simulink model "F16_dynamic_model_2019a"  (R2024b)
settings: Solver=ode3  StartTime=0.0  StopTime=1  FixedStep=1/1000  RelTol=1e-3
values from neighbouring files (symbols this model uses):
  f16data =     [f16aerodata.mat]
  f16engine =     [f16engine.mat]
undefined symbols (not defined in the file or in its folder): e0_0, e1_0, e2_0, e3_0, Earth, ft, m, s, WGS84
libraries: simulink_extras x11, simulink x7, aerosimlib x5, vrlib x3, sharedtransform x3, aerolibfltsims x3, slpidlib x3, aerolibconvert2 x2, aerolibutil x1, sharedutil x1, shared6dof x1, aerolibtransform2 x1
(part 3 of 3)

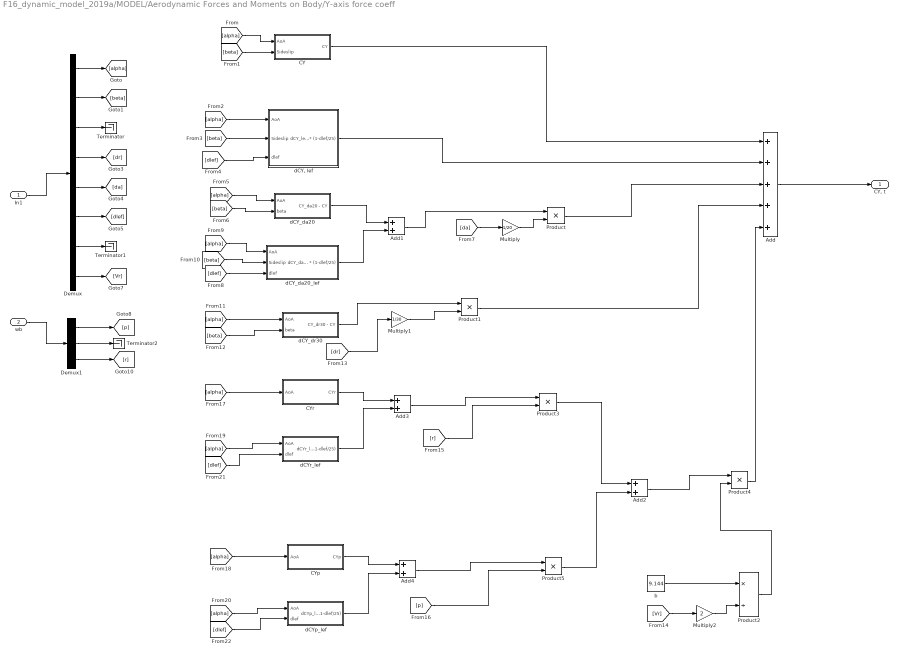
== system F16_dynamic_model_2019a/MODEL/Aerodynamic Forces and Moments on Body/Y-axis force coeff ==
  In1 : Inport
  "wb " : Inport  Port=2
  Add : Sum  Inputs=+++++
  Add{1..4} (4 alike) : Sum
  CY : Subsystem
  CYp : Subsystem
  CYr : Subsystem
  Demux : Demux  Outputs=8
  Demux1 : Demux  Outputs=3
  Multiply : Gain  Gain=1/20
  Multiply1 : Gain  Gain=1/30
  Multiply2 : Gain  Gain=2
  Product{,1,3..5} (5 alike) : Product
  Product2 : Product  Inputs=*/
  Terminator : Terminator
  Terminator1 : Terminator
  Terminator2 : Terminator
  b : Constant  Value=9.144
  "dCY, lef " : Subsystem
  dCY_da20 : Subsystem
  dCY_da20_lef : Subsystem
  dCY_dr30 : Subsystem
  dCYp_lef : Subsystem
  dCYr_lef : Subsystem
  "CY, t" : Outport
  wires:
  Demux/3 -> Terminator/1
  Demux/1 -> [alpha]
  Demux/7 -> Terminator1/1
  Demux/8 -> [Vr]
  Demux/6 -> [dlef]
  Demux/4 -> [dr]
  Demux/2 -> [beta]
  Demux/5 -> [da]
  In1/1 -> Demux/1
  "wb "/1 -> Demux1/1
  Demux1/1 -> [p]
  Demux1/2 -> Terminator2/1
  Demux1/3 -> [r]
  [alpha] -> CY/1(AoA)
  [beta] -> CY/2("Sideslip ")
  Add/1 -> "CY, t"/1
  CY/1(CY) -> Add/1
  [dlef] -> "dCY, lef "/3(dlef)
  [beta] -> "dCY, lef "/2("Sideslip ")
  [alpha] -> "dCY, lef "/1(AoA)
  "dCY, lef "/1(dCY_lef * (1-dlef/25)) -> Add/2
  [alpha] -> dCY_da20/1(AoA)
  [beta] -> dCY_da20/2(beta)
  dCY_da20/1(CY_da20 - CY) -> Add1/1
  Add1/1 -> Product/1
  Product/1 -> Add/3
  [da] -> Multiply/1
  Multiply/1 -> Product/2
  [dlef] -> dCY_da20_lef/3(dlef)
  [beta] -> dCY_da20_lef/2("Sideslip ")
  [alpha] -> dCY_da20_lef/1(AoA)
  dCY_da20_lef/1(dCY_da20lef * (1-dlef/25)) -> Add1/2
  [alpha] -> dCY_dr30/1(AoA)
  [beta] -> dCY_dr30/2(beta)
  dCY_dr30/1(CY_dr30 - CY) -> Product1/1
  [dr] -> Multiply1/1
  Multiply1/1 -> Product1/2
  Product1/1 -> Add/4
  [Vr] -> Multiply2/1
  b/1 -> Product2/1
  Multiply2/1 -> Product2/2
  [r] -> Product3/2
  Product3/1 -> Add2/1
  Add2/1 -> Product4/1
  Product2/1 -> Product4/2
  Product4/1 -> Add/5
  [p] -> Product5/2
  Product5/1 -> Add2/2
  [alpha] -> CYr/1(AoA)
  [alpha] -> dCYr_lef/1(AoA)
  CYr/1(CYr) -> Add3/1
  dCYr_lef/1(dCYr_lef * (1-dlef/25)) -> Add3/2
  Add3/1 -> Product3/1
  CYp/1("CYp ") -> Add4/1
  dCYp_lef/1(dCYp_lef * (1-dlef/25)) -> Add4/2
  Add4/1 -> Product5/1
  [alpha] -> CYp/1(AoA)
  [alpha] -> dCYp_lef/1(AoA)
  [dlef] -> dCYr_lef/2(dlef)
  [dlef] -> dCYp_lef/2(dlef)

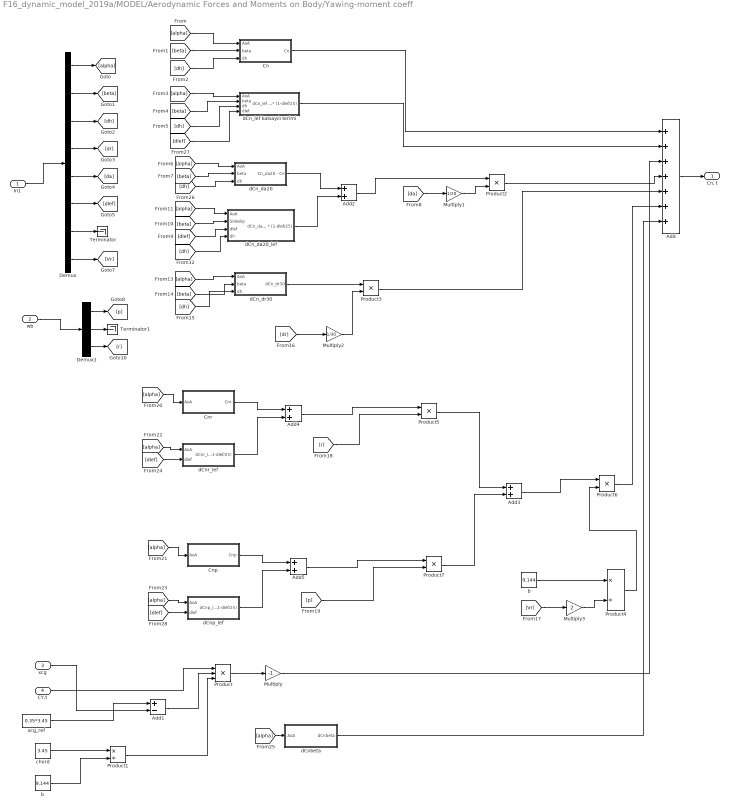
== system F16_dynamic_model_2019a/MODEL/Aerodynamic Forces and Moments on Body/Yawing-moment coeff ==
  In1 : Inport
  wb : Inport  Port=2
  xcg : Inport  Port=3
  CY,t : Inport  Port=4
  Add : Sum  Inputs=+++++++
  Add1 : Sum  Inputs=+-
  Add{2..5} (4 alike) : Sum
  Cn : Subsystem
  Cnp : Subsystem
  Cnr : Subsystem
  Demux : Demux  Outputs=8
  Demux1 : Demux  Outputs=3
  Multiply : Gain  Gain=-1
  Multiply1 : Gain  Gain=1/20
  Multiply2 : Gain  Gain=1/30
  Multiply3 : Gain  Gain=2
  Product : Product  Inputs=3
  Product1 : Product  Inputs=*/
  Product{2..3,5..7} (5 alike) : Product
  Product4 : Product  Inputs=*/
  Terminator : Terminator
  Terminator1 : Terminator
  b : Constant  Value=9.144
  "b " : Constant  Value=9.144
  chord : Constant  Value=3.45
  dCn_da20 : Subsystem
  dCn_da20_lef : Subsystem
  dCn_dr30 : Subsystem
  dCn_lef katsayılı terimi : Subsystem
  dCnbeta : Subsystem
  dCnp_lef : Subsystem
  dCnr_lef : Subsystem
  xcg_ref : Constant  Value=0.35*3.45
  "Cn, t" : Outport
  wires:
  Demux/3 -> [dh]
  Demux/1 -> [alpha]
  Demux/7 -> Terminator/1
  Demux/8 -> [Vr]
  Demux/6 -> [dlef]
  Demux/4 -> [dr]
  Demux/2 -> [beta]
  Demux/5 -> [da]
  In1/1 -> Demux/1
  wb/1 -> Demux1/1
  Demux1/1 -> [p]
  Demux1/2 -> Terminator1/1
  Demux1/3 -> [r]
  [alpha] -> Cn/1(AoA)
  [beta] -> Cn/2("beta ")
  [dh] -> Cn/3(dh)
  [alpha] -> dCn_lef katsayılı terimi/1(AoA)
  [beta] -> dCn_lef katsayılı terimi/2(beta)
  [dh] -> dCn_lef katsayılı terimi/3(dh)
  Cn/1(Cn) -> Add/1
  dCn_lef katsayılı terimi/1(dCn_lef * (1-dlef/25)) -> Add/2
  CY,t/1 -> Product/1
  xcg_ref/1 -> Add1/1
  xcg/1 -> Add1/2
  Add1/1 -> Product/2
  chord/1 -> Product1/1
  "b "/1 -> Product1/2
  Product1/1 -> Product/3
  Product/1 -> Multiply/1
  Multiply/1 -> Add/3
  Add/1 -> "Cn, t"/1
  Add2/1 -> Product2/1
  [beta] -> dCn_da20_lef/2("Sideslip ")
  dCn_da20_lef/1(dCn_da20lef * (1-dlef/25)) -> Add2/2
  dCn_da20/1(Cn_da20 - Cn) -> Add2/1
  [alpha] -> dCn_da20_lef/1(AoA)
  Product2/1 -> Add/4
  Multiply1/1 -> Product2/2
  [da] -> Multiply1/1
  [alpha] -> dCn_da20/1(AoA)
  [dlef] -> dCn_da20_lef/3(dlef)
  [beta] -> dCn_da20/2(beta)
  [dh] -> dCn_da20_lef/4(dh)
  [alpha] -> dCn_dr30/1(AoA)
  [beta] -> dCn_dr30/2(beta)
  [dh] -> dCn_dr30/3(dh)
  [dr] -> Multiply2/1
  Multiply2/1 -> Product3/2
  dCn_dr30/1(dCn_dr30) -> Product3/1
  Product3/1 -> Add/5
  b/1 -> Product4/1
  Product7/1 -> Add3/2
  Add3/1 -> Product6/1
  [alpha] -> dCnp_lef/1(AoA)
  [alpha] -> Cnp/1(AoA)
  Add5/1 -> Product7/1
  Cnp/1("Cnp ") -> Add5/1
  dCnp_lef/1(dCnp_lef * (1-dlef/25)) -> Add5/2
  dCnr_lef/1(dCnr_lef * (1-dlef/25)) -> Add4/2
  [Vr] -> Multiply3/1
  Multiply3/1 -> Product4/2
  Cnr/1(Cnr) -> Add4/1
  Add4/1 -> Product5/1
  [alpha] -> Cnr/1(AoA)
  [alpha] -> dCnr_lef/1(AoA)
  Product6/1 -> Add/6
  [r] -> Product5/2
  [p] -> Product7/2
  Product5/1 -> Add3/1
  Product4/1 -> Product6/2
  [dlef] -> dCnr_lef/2(dlef)
  [alpha] -> dCnbeta/1(AoA)
  dCnbeta/1("dCnbeta ") -> Add/7
  [dh] -> dCn_da20/3(dh)
  [dlef] -> dCn_lef katsayılı terimi/4(dlef)
  [dlef] -> dCnp_lef/2(dlef)

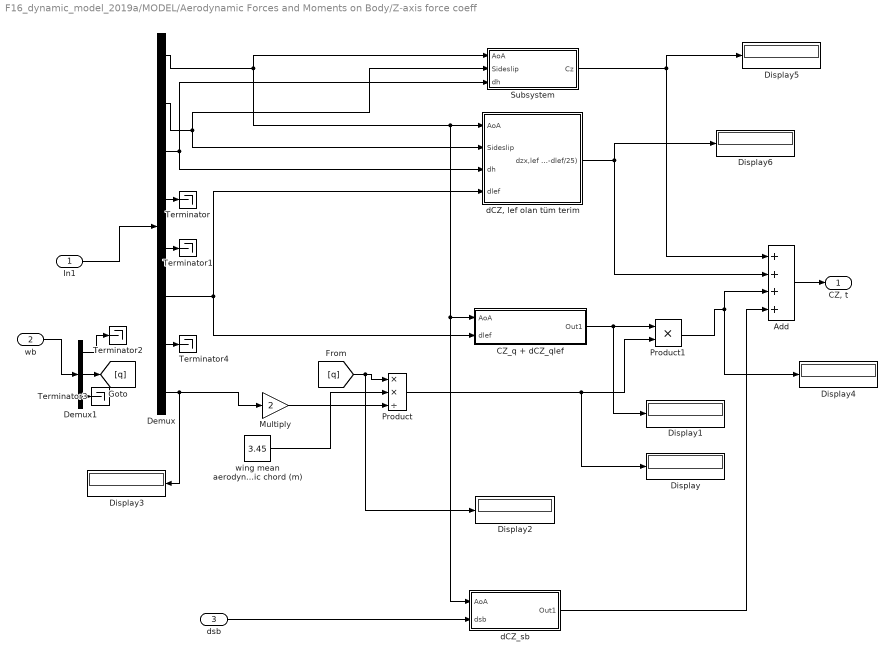
== system F16_dynamic_model_2019a/MODEL/Aerodynamic Forces and Moments on Body/Z-axis force coeff ==
  In1 : Inport
  wb : Inport  Port=2
  dsb : Inport  Port=3
  Add : Sum  Inputs=++++
  CZ_q + dCZ_qlef : Subsystem
  Demux : Demux  Outputs=8
  Demux1 : Demux  Outputs=3
  Display{,1..6} (7 alike) : Display
  Multiply : Gain  Gain=2
  Product : Product  Inputs=**/
  Product1 : Product
  Subsystem : Subsystem
  Terminator{,1..4} (5 alike) : Terminator
  "dCZ, lef olan tüm terim" : Subsystem
  dCZ_sb : Subsystem
  wing mean aerodynamic chord (m) : Constant  Value=3.45
  "CZ, t" : Outport
  wires:
  Product1/1 -> Display4/1, Add/3
  Product/1 -> Display/1, Product1/2
  Multiply/1 -> Product/3
  wing mean aerodynamic chord (m)/1 -> Product/2
  Demux/8 -> Multiply/1, Display3/1
  Demux/5 -> Terminator1/1
  Demux/4 -> Terminator/1
  CZ_q + dCZ_qlef/1(Out1) -> Display1/1, Product1/1
  Demux/6 -> "dCZ, lef olan tüm terim"/4(dlef), CZ_q + dCZ_qlef/2(dlef)
  Demux/3 -> Subsystem/3(dh), "dCZ, lef olan tüm terim"/3(dh)
  Demux/2 -> "dCZ, lef olan tüm terim"/2("Sideslip "), Subsystem/2(Sideslip)
  Demux/1 -> Subsystem/1(AoA), "dCZ, lef olan tüm terim"/1(AoA), dCZ_sb/1(AoA), CZ_q + dCZ_qlef/1(AoA)
  "dCZ, lef olan tüm terim"/1(dzx,lef * (1-dlef/25)) -> Add/2, Display6/1
  Subsystem/1(Cz) -> Add/1, Display5/1
  Add/1 -> "CZ, t"/1
  In1/1 -> Demux/1
  Demux1/2 -> [q]
  Demux1/1 -> Terminator2/1
  wb/1 -> Demux1/1
  Demux1/3 -> Terminator3/1
  [q] -> Display2/1, Product/1
  Demux/7 -> Terminator4/1
  dsb/1 -> dCZ_sb/2(dsb)
  dCZ_sb/1(Out1) -> Add/4

== system F16_dynamic_model_2019a/MODEL/Thrust on Body /Subsystem ==
  Mil : Inport
  Idle : Inport  Port=2
  power : Inport  Port=3
  Max : Inport  Port=4
  Display : Display
  Display1 : Display
  Display2 : Display
  Multiply : Gain  Gain=4.448
  Subsystem : Subsystem
  Subsystem1 : Subsystem
  Switch : Switch  Criteria=u2 > Threshold  Threshold=50  SaturateOnIntegerOverflow=off  InputSameDT=off
  Thrust : Outport
  wires:
  Mil/1 -> [T_Mil]
  Idle/1 -> [T_Idle]
  [T_Mil] -> Subsystem/1(mil)
  [T_Max] -> Subsystem/2("max ")
  Max/1 -> [T_Max]
  power/1 -> Display2/1, [Power]
  [Power] -> Subsystem/3(power)
  Subsystem/1(T) -> Display/1, Switch/1
  [Power] -> Switch/2
  [T_Mil] -> Subsystem1/1("Mil ")
  Subsystem1/1(T) -> Switch/3, Display1/1
  Switch/1 -> Multiply/1
  [T_Idle] -> Subsystem1/2(Idle)
  [Power] -> Subsystem1/3(Power)
  Multiply/1 -> Thrust/1

== system F16_dynamic_model_2019a/MODEL/gravity/gravity_body_axis ==
  gravity : Inport
  "phi theta psi " : Inport  Port=2
  Demux : Demux  Outputs=3
  Gain : Gain  Gain=-1
  Mux : Mux  Inputs=3
  Product : Product
  Product1 : Product
  Product2 : Product
  SinCos : Trigonometry  Operator=sincos
  SinCos1 : Trigonometry  Operator=sincos
  Terminator : Terminator
  gravity_body : Outport
  wires:
  Demux/1 -> SinCos/1
  Demux/2 -> SinCos1/1
  SinCos/1 -> Product/1
  SinCos1/2 -> Product/2, Product1/2
  Product/1 -> Mux/2
  SinCos/2 -> Product1/1
  Product1/1 -> Mux/3
  SinCos1/1 -> Gain/1
  Gain/1 -> Mux/1
  gravity/1 -> Product2/1
  Mux/1 -> Product2/2
  Product2/1 -> gravity_body/1
  "phi theta psi "/1 -> Demux/1
  Demux/3 -> Terminator/1

== system F16_dynamic_model_2019a/MODEL/6-DOF Model Body Euler/Subsystem/Subsystem ==
  p q r : Inport
  q0 q1 q2 q3 : Inport  Port=2
  Constant : Constant
  Dot Product : DotProduct  InputSameDT=off  OutDataTypeStr=Inherit: Inherit via internal rule
  High Gain Quaternion Normalization : Gain  SaturateOnIntegerOverflow=on  OutDataTypeStr=Inherit: Same as input  ParamDataTypeStr=Inherit: Same as input
  Mux1 : Mux  Inputs=[3 4 1]
  Mux2 : Mux
  Sum : Sum  Inputs=|+-  InputSameDT=on  SaturateOnIntegerOverflow=on  OutDataTypeStr=Inherit: Same as first input
  q0dot : Fcn  Expr=-0.5 * ( u[5]*u[1]+u[6]*u[2]+u[7]*u[3] ) + u[8]*u[4]
  q1dot : Fcn  Expr=0.5 * ( u[4]*u[1]+u[6]*u[3]-u[7]*u[2] ) + u[8]*u[5]
  q2dot : Fcn  Expr=0.5 * ( u[4]*u[2]+u[7]*u[1]-u[5]*u[3] ) + u[8]*u[6]
  q3dot : Fcn  Expr=0.5 * ( u[4]*u[3]+u[5]*u[2]-u[6]*u[1] ) + u[8]*u[7]
  qdot : Outport  InitialOutput=0  VectorParamsAs1DForOutWhenUnconnected=off
  wires:
  q0 q1 q2 q3/1 -> Dot Product/1, Dot Product/2, Mux1/2
  q3dot/1 -> Mux2/4
  Mux2/1 -> qdot/1
  Mux1/1 -> q2dot/1, q3dot/1, q0dot/1, q1dot/1
  Sum/1 -> High Gain Quaternion Normalization/1
  q1dot/1 -> Mux2/2
  Dot Product/1 -> Sum/2
  High Gain Quaternion Normalization/1 -> Mux1/3
  q0dot/1 -> Mux2/1
  Constant/1 -> Sum/1
  p q r/1 -> Mux1/1
  q2dot/1 -> Mux2/3

== system F16_dynamic_model_2019a/MODEL/Aerodynamic Forces and Moments on Body/Pitching-moment coeff/Cm ==
  AoA : Inport
  beta : Inport  Port=2
  dh : Inport  Port=3
  n-D Lookup Table : Lookup_n-D  NumberOfTableDimensions=3  BreakpointsForDimension1=f16data.alpha1  BreakpointsForDimension2=f16data.beta  BreakpointsForDimension3=f16data.de1  Table=f16data.Cm  InterpMethod=Cubic spline  ExtrapMethod=Clip  InternalRulePriority=Speed  RndMeth=Simplest
      settings: InputPortMap=u0,u1,u2
  Cm : Outport
  wires:
  n-D Lookup Table/1 -> Cm/1
  beta/1 -> n-D Lookup Table/2
  AoA/1 -> n-D Lookup Table/1
  dh/1 -> n-D Lookup Table/3

== system F16_dynamic_model_2019a/MODEL/Aerodynamic Forces and Moments on Body/Pitching-moment coeff/Cm_q - dCm_qlef ==
  AoA : Inport
  dlef : Inport  Port=2
  Add : Sum
  Cmq : Lookup_n-D  NumberOfTableDimensions=1  BreakpointsForDimension1=f16data.alpha1  BreakpointsForDimension3=[5, 7]  Table=f16data.Cmq  ExtrapMethod=Clip  InternalRulePriority=Speed  RndMeth=Simplest
  Constant : Constant
  Display : Display
  Multiply : Gain  Gain=1/(25)
  Product : Product
  Sum : Sum  Inputs=+-
  dCmq_lef : Lookup_n-D  NumberOfTableDimensions=1  BreakpointsForDimension1=f16data.alpha2  BreakpointsForDimension3=[5, 7]  Table=f16data.dCmq_lef  ExtrapMethod=Clip  InternalRulePriority=Speed  RndMeth=Simplest
  Out1 : Outport
  wires:
  Multiply/1 -> Sum/2
  Constant/1 -> Sum/1
  Sum/1 -> Product/2
  dlef/1 -> Multiply/1
  Product/1 -> Add/2
  AoA/1 -> Cmq/1, dCmq_lef/1
  Cmq/1 -> Display/1, Add/1
  dCmq_lef/1 -> Product/1
  Add/1 -> Out1/1

== system F16_dynamic_model_2019a/MODEL/Aerodynamic Forces and Moments on Body/Pitching-moment coeff/dCm ==
  AoA : Inport
  n-D Lookup Table : Lookup_n-D  NumberOfTableDimensions=1  BreakpointsForDimension1=f16data.alpha1  BreakpointsForDimension3=[5, 7]  Table=f16data.dCm  ExtrapMethod=Clip  InternalRulePriority=Speed  RndMeth=Simplest
  dCm : Outport
  wires:
  n-D Lookup Table/1 -> dCm/1
  AoA/1 -> n-D Lookup Table/1

== system F16_dynamic_model_2019a/MODEL/Aerodynamic Forces and Moments on Body/Pitching-moment coeff/dCm, lef olan tüm terim ==
  AoA : Inport
  "Sideslip " : Inport  Port=2
  dh : Inport  Port=3
  dlef : Inport  Port=4
  Cm : Lookup_n-D  NumberOfTableDimensions=3  BreakpointsForDimension1=f16data.alpha1  BreakpointsForDimension2=f16data.beta  BreakpointsForDimension3=f16data.de1  Table=f16data.Cm  ExtrapMethod=Clip  InternalRulePriority=Speed  RndMeth=Simplest
      settings: InputPortMap=u0,u1,u2
  Cm_lef : Lookup_n-D  BreakpointsForDimension1=f16data.alpha2  BreakpointsForDimension2=f16data.beta  BreakpointsForDimension3=[5, 7]  Table=f16data.Cm_lef  ExtrapMethod=Clip  InternalRulePriority=Speed  RndMeth=Simplest
      settings: InputPortMap=u0,u1
  Constant : Constant
  Multiply : Gain  Gain=1/(25)
  Multiply1 : Gain  Gain=0
  Product : Product
  Sum : Sum  Inputs=+-
  dcm,lef : Sum  Inputs=+-
  dcm,lef * (1-dlef/25) : Outport
  wires:
  dlef/1 -> Multiply/1
  Multiply/1 -> Sum/2
  Constant/1 -> Sum/1
  Sum/1 -> Product/2
  dh/1 -> Multiply1/1
  dcm,lef/1 -> Product/1
  Product/1 -> dcm,lef * (1-dlef/25)/1
  Cm/1 -> dcm,lef/2
  Cm_lef/1 -> dcm,lef/1
  AoA/1 -> Cm/1, Cm_lef/1
  "Sideslip "/1 -> Cm/2, Cm_lef/2
  Multiply1/1 -> Cm/3

== system F16_dynamic_model_2019a/MODEL/Aerodynamic Forces and Moments on Body/Pitching-moment coeff/dCm_ds ==
  AoA : Inport
  dh : Inport  Port=2
  n-D Lookup Table : Lookup_n-D  BreakpointsForDimension1=f16data.alpha1  BreakpointsForDimension2=f16data.de3  BreakpointsForDimension3=[5, 7]  Table=f16data.dCm_ds  ExtrapMethod=Clip  InternalRulePriority=Speed  RndMeth=Simplest
      settings: InputPortMap=u0,u1
  dCm_ds : Outport
  wires:
  n-D Lookup Table/1 -> dCm_ds/1
  dh/1 -> n-D Lookup Table/2
  AoA/1 -> n-D Lookup Table/1

== system F16_dynamic_model_2019a/MODEL/Aerodynamic Forces and Moments on Body/Pitching-moment coeff/dCm_sb ==
  AoA : Inport
  dsb : Inport  Port=2
  Multiply : Gain  Gain=1/60
  Product : Product
  n-D Lookup Table : Lookup_n-D  NumberOfTableDimensions=1  BreakpointsForDimension1=f16data.alpha1  BreakpointsForDimension3=[5, 7]  Table=f16data.dCm_sb  ExtrapMethod=Clip  InternalRulePriority=Speed  RndMeth=Simplest
  Out1 : Outport
  wires:
  dsb/1 -> Multiply/1
  AoA/1 -> n-D Lookup Table/1
  n-D Lookup Table/1 -> Product/1
  Multiply/1 -> Product/2
  Product/1 -> Out1/1

== system F16_dynamic_model_2019a/MODEL/Aerodynamic Forces and Moments on Body/Rolling-moment coeff/Cl ==
  AoA : Inport
  "beta " : Inport  Port=2
  dh : Inport  Port=3
  Cl table : Lookup_n-D  NumberOfTableDimensions=3  BreakpointsForDimension1=f16data.alpha1  BreakpointsForDimension2=f16data.beta  BreakpointsForDimension3=f16data.de2  Table=f16data.Cl  ExtrapMethod=Clip  InternalRulePriority=Speed  RndMeth=Simplest
      settings: InputPortMap=u0,u1,u2
  Cl : Outport
  wires:
  AoA/1 -> Cl table/1
  "beta "/1 -> Cl table/2
  dh/1 -> Cl table/3
  Cl table/1 -> Cl/1

== system F16_dynamic_model_2019a/MODEL/Aerodynamic Forces and Moments on Body/Rolling-moment coeff/Clp ==
  AoA : Inport
  Clp : Lookup_n-D  NumberOfTableDimensions=1  BreakpointsForDimension1=f16data.alpha1  BreakpointsForDimension3=[5, 7]  Table=f16data.Clp  ExtrapMethod=Clip  InternalRulePriority=Speed  RndMeth=Simplest
  "Clp " : Outport
  wires:
  AoA/1 -> Clp/1
  Clp/1 -> "Clp "/1

== system F16_dynamic_model_2019a/MODEL/Aerodynamic Forces and Moments on Body/Rolling-moment coeff/Clr ==
  AoA : Inport
  n-D Lookup Table : Lookup_n-D  NumberOfTableDimensions=1  BreakpointsForDimension1=f16data.alpha1  BreakpointsForDimension3=[5, 7]  Table=f16data.Clr  ExtrapMethod=Clip  InternalRulePriority=Speed  RndMeth=Simplest
  Clr : Outport
  wires:
  AoA/1 -> n-D Lookup Table/1
  n-D Lookup Table/1 -> Clr/1

== system F16_dynamic_model_2019a/MODEL/Aerodynamic Forces and Moments on Body/Rolling-moment coeff/dCl_da20 ==
  AoA : Inport
  beta : Inport  Port=2
  dh : Inport  Port=3
  Add : Sum  Inputs=+-
  Cl : Lookup_n-D  NumberOfTableDimensions=3  BreakpointsForDimension1=f16data.alpha1  BreakpointsForDimension2=f16data.beta  BreakpointsForDimension3=f16data.de2  Table=f16data.Cl  ExtrapMethod=Clip  InternalRulePriority=Speed  RndMeth=Simplest
      settings: InputPortMap=u0,u1,u2
  Cl_da20 : Lookup_n-D  BreakpointsForDimension1=f16data.alpha1  BreakpointsForDimension2=f16data.beta  BreakpointsForDimension3=[5, 7]  Table=f16data.Cl_da20  ExtrapMethod=Clip  InternalRulePriority=Speed  RndMeth=Simplest
      settings: InputPortMap=u0,u1
  Multiply : Gain  Gain=0
  Cl_da20 - Cl : Outport
  wires:
  AoA/1 -> Cl/1, Cl_da20/1
  beta/1 -> Cl/2, Cl_da20/2
  Cl_da20/1 -> Add/1
  Cl/1 -> Add/2
  Add/1 -> Cl_da20 - Cl/1
  dh/1 -> Multiply/1
  Multiply/1 -> Cl/3

== system F16_dynamic_model_2019a/MODEL/Aerodynamic Forces and Moments on Body/Rolling-moment coeff/dCl_da20_lef katsayılı terim ==
  AoA : Inport
  "Sideslip " : Inport  Port=2
  dlef : Inport  Port=3
  dh : Inport  Port=4
  Add : Sum  Inputs=+-
  Cl table : Lookup_n-D  NumberOfTableDimensions=3  BreakpointsForDimension1=f16data.alpha1  BreakpointsForDimension2=f16data.beta  BreakpointsForDimension3=f16data.de2  Table=f16data.Cl  ExtrapMethod=Clip  InternalRulePriority=Speed  RndMeth=Simplest
      settings: InputPortMap=u0,u1,u2
  Cl_da20 : Lookup_n-D  BreakpointsForDimension1=f16data.alpha1  BreakpointsForDimension2=f16data.beta  BreakpointsForDimension3=[5, 7]  Table=f16data.Cl_da20  ExtrapMethod=Clip  InternalRulePriority=Speed  RndMeth=Simplest
      settings: InputPortMap=u0,u1
  Cl_da20lef : Lookup_n-D  BreakpointsForDimension1=f16data.alpha2  BreakpointsForDimension2=f16data.beta  BreakpointsForDimension3=[5, 7]  Table=f16data.Cl_da20lef  ExtrapMethod=Clip  InternalRulePriority=Speed  RndMeth=Simplest
      settings: InputPortMap=u0,u1
  Cl_lef : Lookup_n-D  BreakpointsForDimension1=f16data.alpha2  BreakpointsForDimension2=f16data.beta  BreakpointsForDimension3=[5, 7]  Table=f16data.Cl_lef  ExtrapMethod=Clip  InternalRulePriority=Speed  RndMeth=Simplest
      settings: InputPortMap=u0,u1
  Constant : Constant
  Multiply : Gain  Gain=1/(25)
  Multiply1 : Gain  Gain=0
  Product : Product
  Sum : Sum  Inputs=+-
  dCl_da20lef : Sum  Inputs=+--
  dCl_da20lef * (1-dlef/25) : Outport
  wires:
  "Sideslip "/1 -> Cl table/2, Cl_da20/2, Cl_lef/2, Cl_da20lef/2
  AoA/1 -> Cl table/1, Cl_da20/1, Cl_lef/1, Cl_da20lef/1
  Constant/1 -> Sum/1
  Cl_lef/1 -> dCl_da20lef/2
  dlef/1 -> Multiply/1
  Multiply/1 -> Sum/2
  dCl_da20lef/1 -> Product/1
  Product/1 -> dCl_da20lef * (1-dlef/25)/1
  Cl_da20lef/1 -> dCl_da20lef/1
  Sum/1 -> Product/2
  Cl_da20/1 -> Add/1
  Cl table/1 -> Add/2
  Add/1 -> dCl_da20lef/3
  dh/1 -> Multiply1/1
  Multiply1/1 -> Cl table/3

== system F16_dynamic_model_2019a/MODEL/Aerodynamic Forces and Moments on Body/Rolling-moment coeff/dCl_dr30 ==
  AoA : Inport
  beta : Inport  Port=2
  dh : Inport  Port=3
  Add : Sum  Inputs=+-
  Cl table : Lookup_n-D  NumberOfTableDimensions=3  BreakpointsForDimension1=f16data.alpha1  BreakpointsForDimension2=f16data.beta  BreakpointsForDimension3=f16data.de2  Table=f16data.Cl  ExtrapMethod=Clip  InternalRulePriority=Speed  RndMeth=Simplest
      settings: InputPortMap=u0,u1,u2
  Cl_dr30 : Lookup_n-D  BreakpointsForDimension1=f16data.alpha1  BreakpointsForDimension2=f16data.beta  BreakpointsForDimension3=[5, 7]  Table=f16data.Cl_dr30  ExtrapMethod=Clip  InternalRulePriority=Speed  RndMeth=Simplest
      settings: InputPortMap=u0,u1
  Multiply : Gain  Gain=0
  dCl_dr30 : Outport
  wires:
  Cl_dr30/1 -> Add/1
  dh/1 -> Multiply/1
  AoA/1 -> Cl table/1, Cl_dr30/1
  Add/1 -> dCl_dr30/1
  Cl table/1 -> Add/2
  beta/1 -> Cl_dr30/2, Cl table/2
  Multiply/1 -> Cl table/3

== system F16_dynamic_model_2019a/MODEL/Aerodynamic Forces and Moments on Body/Rolling-moment coeff/dCl_lef katsayılı terimi ==
  AoA : Inport
  beta : Inport  Port=2
  dh : Inport  Port=3
  dlef : Inport  Port=4
  Add : Sum  Inputs=+-
  Cl table : Lookup_n-D  NumberOfTableDimensions=3  BreakpointsForDimension1=f16data.alpha1  BreakpointsForDimension2=f16data.beta  BreakpointsForDimension3=f16data.de2  Table=f16data.Cl  ExtrapMethod=Clip  InternalRulePriority=Speed  RndMeth=Simplest
      settings: InputPortMap=u0,u1,u2
  Cl_lef : Lookup_n-D  BreakpointsForDimension1=f16data.alpha2  BreakpointsForDimension2=f16data.beta  BreakpointsForDimension3=[5, 7]  Table=f16data.Cl_lef  ExtrapMethod=Clip  InternalRulePriority=Speed  RndMeth=Simplest
      settings: InputPortMap=u0,u1
  Constant : Constant
  Multiply : Gain  Gain=0
  Multiply1 : Gain  Gain=1/(25)
  Product : Product
  Sum : Sum  Inputs=+-
  dCl_lef * (1-dlef/25) : Outport
  wires:
  AoA/1 -> Cl table/1, Cl_lef/1
  beta/1 -> Cl_lef/2, Cl table/2
  dh/1 -> Multiply/1
  Multiply/1 -> Cl table/3
  Cl_lef/1 -> Add/1
  Cl table/1 -> Add/2
  Constant/1 -> Sum/1
  Multiply1/1 -> Sum/2
  Sum/1 -> Product/2
  dlef/1 -> Multiply1/1
  Add/1 -> Product/1
  Product/1 -> dCl_lef * (1-dlef/25)/1

== system F16_dynamic_model_2019a/MODEL/Aerodynamic Forces and Moments on Body/Rolling-moment coeff/dClbeta ==
  AoA : Inport
  n-D Lookup Table : Lookup_n-D  NumberOfTableDimensions=1  BreakpointsForDimension1=f16data.alpha1  BreakpointsForDimension3=[5, 7]  Table=f16data.dClbeta  ExtrapMethod=Clip  InternalRulePriority=Speed  RndMeth=Simplest
  "dClbeta " : Outport
  wires:
  AoA/1 -> n-D Lookup Table/1
  n-D Lookup Table/1 -> "dClbeta "/1

== system F16_dynamic_model_2019a/MODEL/Aerodynamic Forces and Moments on Body/Rolling-moment coeff/dClp_lef ==
  AoA : Inport
  dlef : Inport  Port=2
  Constant : Constant
  Multiply : Gain  Gain=1/(25)
  Product : Product
  Sum : Sum  Inputs=+-
  dClp_lef : Lookup_n-D  NumberOfTableDimensions=1  BreakpointsForDimension1=f16data.alpha2  BreakpointsForDimension3=[5, 7]  Table=f16data.dClp_lef  ExtrapMethod=Clip  InternalRulePriority=Speed  RndMeth=Simplest
  dClp_lef * (1-dlef/25) : Outport
  wires:
  AoA/1 -> dClp_lef/1
  Constant/1 -> Sum/1
  dlef/1 -> Multiply/1
  Multiply/1 -> Sum/2
  Product/1 -> dClp_lef * (1-dlef/25)/1
  Sum/1 -> Product/2
  dClp_lef/1 -> Product/1

== system F16_dynamic_model_2019a/MODEL/Aerodynamic Forces and Moments on Body/Rolling-moment coeff/dClr_lef ==
  AoA : Inport
  dlef : Inport  Port=2
  Constant : Constant
  Multiply : Gain  Gain=1/(25)
  Product : Product
  Sum : Sum  Inputs=+-
  dClr_lef : Lookup_n-D  NumberOfTableDimensions=1  BreakpointsForDimension1=f16data.alpha2  BreakpointsForDimension3=[5, 7]  Table=f16data.dClr_lef  ExtrapMethod=Clip  InternalRulePriority=Speed  RndMeth=Simplest
  dClr_lef * (1-dlef/25) : Outport
  wires:
  AoA/1 -> dClr_lef/1
  Constant/1 -> Sum/1
  dlef/1 -> Multiply/1
  Multiply/1 -> Sum/2
  Product/1 -> dClr_lef * (1-dlef/25)/1
  Sum/1 -> Product/2
  dClr_lef/1 -> Product/1

== system F16_dynamic_model_2019a/MODEL/Aerodynamic Forces and Moments on Body/X-axis force coeff/CX_q - dCX_qlef ==
  AoA : Inport
  dlef : Inport  Port=2
  Add : Sum
  CXq : Lookup_n-D  NumberOfTableDimensions=1  BreakpointsForDimension1=f16data.alpha1  BreakpointsForDimension3=[5, 7]  Table=f16data.CXq  ExtrapMethod=Clip  InternalRulePriority=Speed  RndMeth=Simplest
  Constant : Constant
  Multiply : Gain  Gain=1/(25)
  Product : Product
  Sum : Sum  Inputs=+-
  dCXq_lef : Lookup_n-D  NumberOfTableDimensions=1  BreakpointsForDimension1=f16data.alpha2  BreakpointsForDimension3=[5, 7]  Table=f16data.dCXq_lef  ExtrapMethod=Clip  InternalRulePriority=Speed  RndMeth=Simplest
  Out1 : Outport
  wires:
  Multiply/1 -> Sum/2
  Constant/1 -> Sum/1
  Sum/1 -> Product/2
  dlef/1 -> Multiply/1
  Product/1 -> Add/2
  AoA/1 -> dCXq_lef/1, CXq/1
  CXq/1 -> Add/1
  dCXq_lef/1 -> Product/1
  Add/1 -> Out1/1

== system F16_dynamic_model_2019a/MODEL/Aerodynamic Forces and Moments on Body/X-axis force coeff/Subsystem ==
  AoA : Inport
  Sideslip : Inport  Port=2
  dh : Inport  Port=3
  CX : Lookup_n-D  NumberOfTableDimensions=3  BreakpointsForDimension1=f16data.alpha1  BreakpointsForDimension2=f16data.beta  BreakpointsForDimension3=f16data.de1  Table=f16data.CX  ExtrapMethod=Clip  InternalRulePriority=Speed  RndMeth=Simplest
      settings: InputPortMap=u0,u1,u2
  Cx : Outport
  wires:
  AoA/1 -> CX/1
  Sideslip/1 -> CX/2
  dh/1 -> CX/3
  CX/1 -> Cx/1

== system F16_dynamic_model_2019a/MODEL/Aerodynamic Forces and Moments on Body/X-axis force coeff/dCX, lef olan tüm terim ==
  AoA : Inport
  "Sideslip " : Inport  Port=2
  dh : Inport  Port=3
  dlef : Inport  Port=4
  CX : Lookup_n-D  NumberOfTableDimensions=3  BreakpointsForDimension1=f16data.alpha1  BreakpointsForDimension2=f16data.beta  BreakpointsForDimension3=f16data.de1  Table=f16data.CX  ExtrapMethod=Clip  InternalRulePriority=Speed  RndMeth=Simplest
      settings: InputPortMap=u0,u1,u2
  CX_lef : Lookup_n-D  BreakpointsForDimension1=f16data.alpha2  BreakpointsForDimension2=f16data.beta  BreakpointsForDimension3=[5, 7]  Table=f16data.CX_lef  ExtrapMethod=Clip  InternalRulePriority=Speed  RndMeth=Simplest
      settings: InputPortMap=u0,u1
  Constant : Constant
  Multiply : Gain  Gain=1/(25)
  Multiply1 : Gain  Gain=0
  Product : Product
  Sum : Sum  Inputs=+-
  dcx,lef : Sum  Inputs=+-
  dcx,lef * (1-dlef/25) : Outport
  wires:
  dlef/1 -> Multiply/1
  Multiply/1 -> Sum/2
  Constant/1 -> Sum/1
  Sum/1 -> Product/2
  CX/1 -> dcx,lef/2
  CX_lef/1 -> dcx,lef/1
  dh/1 -> Multiply1/1
  dcx,lef/1 -> Product/1
  Product/1 -> dcx,lef * (1-dlef/25)/1
  AoA/1 -> CX/1, CX_lef/1
  "Sideslip "/1 -> CX/2, CX_lef/2
  Multiply1/1 -> CX/3

== system F16_dynamic_model_2019a/MODEL/Aerodynamic Forces and Moments on Body/X-axis force coeff/dCX_sb ==
  AoA : Inport
  dsb : Inport  Port=2
  Multiply : Gain  Gain=1/60
  Product : Product
  n-D Lookup Table : Lookup_n-D  NumberOfTableDimensions=1  BreakpointsForDimension1=f16data.alpha1  BreakpointsForDimension3=[5, 7]  Table=f16data.dCX_sb  ExtrapMethod=Clip  InternalRulePriority=Speed  RndMeth=Simplest
  Out1 : Outport
  wires:
  dsb/1 -> Multiply/1
  AoA/1 -> n-D Lookup Table/1
  n-D Lookup Table/1 -> Product/1
  Multiply/1 -> Product/2
  Product/1 -> Out1/1

== system F16_dynamic_model_2019a/MODEL/Aerodynamic Forces and Moments on Body/Y-axis force coeff/CY ==
  AoA : Inport
  "Sideslip " : Inport  Port=2
  n-D Lookup Table : Lookup_n-D  BreakpointsForDimension1=f16data.alpha1  BreakpointsForDimension2=f16data.beta  BreakpointsForDimension3=[5, 7]  Table=f16data.CY  ExtrapMethod=Clip  InternalRulePriority=Speed  RndMeth=Simplest
      settings: InputPortMap=u0,u1
  CY : Outport
  wires:
  AoA/1 -> n-D Lookup Table/1
  "Sideslip "/1 -> n-D Lookup Table/2
  n-D Lookup Table/1 -> CY/1

== system F16_dynamic_model_2019a/MODEL/Aerodynamic Forces and Moments on Body/Y-axis force coeff/CYp ==
  AoA : Inport
  CYp : Lookup_n-D  NumberOfTableDimensions=1  BreakpointsForDimension1=f16data.alpha1  BreakpointsForDimension3=[5, 7]  Table=f16data.CYp  ExtrapMethod=Clip  InternalRulePriority=Speed  RndMeth=Simplest
  "CYp " : Outport
  wires:
  AoA/1 -> CYp/1
  CYp/1 -> "CYp "/1

== system F16_dynamic_model_2019a/MODEL/Aerodynamic Forces and Moments on Body/Y-axis force coeff/CYr ==
  AoA : Inport
  n-D Lookup Table : Lookup_n-D  NumberOfTableDimensions=1  BreakpointsForDimension1=f16data.alpha1  BreakpointsForDimension3=[5, 7]  Table=f16data.CYr  ExtrapMethod=Clip  InternalRulePriority=Speed  RndMeth=Simplest
  CYr : Outport
  wires:
  AoA/1 -> n-D Lookup Table/1
  n-D Lookup Table/1 -> CYr/1

== system F16_dynamic_model_2019a/MODEL/Aerodynamic Forces and Moments on Body/Y-axis force coeff/dCY, lef  ==
  AoA : Inport
  "Sideslip " : Inport  Port=2
  dlef : Inport  Port=3
  CY : Lookup_n-D  BreakpointsForDimension1=f16data.alpha1  BreakpointsForDimension2=f16data.beta  BreakpointsForDimension3=[5, 7]  Table=f16data.CY  ExtrapMethod=Clip  InternalRulePriority=Speed  RndMeth=Simplest
      settings: InputPortMap=u0,u1
  Constant : Constant
  Multiply : Gain  Gain=1/(25)
  Product : Product
  Sum : Sum  Inputs=+-
  dCY_lef : Lookup_n-D  BreakpointsForDimension1=f16data.alpha2  BreakpointsForDimension2=f16data.beta  BreakpointsForDimension3=[5, 7]  Table=f16data.CY_lef  ExtrapMethod=Clip  InternalRulePriority=Speed  RndMeth=Simplest
      settings: InputPortMap=u0,u1
  dcy,lef : Sum  Inputs=+-
  dCY_lef * (1-dlef/25) : Outport
  wires:
  Product/1 -> dCY_lef * (1-dlef/25)/1
  dcy,lef/1 -> Product/1
  dCY_lef/1 -> dcy,lef/1
  CY/1 -> dcy,lef/2
  Sum/1 -> Product/2
  Constant/1 -> Sum/1
  Multiply/1 -> Sum/2
  dlef/1 -> Multiply/1
  AoA/1 -> CY/1, dCY_lef/1
  "Sideslip "/1 -> CY/2, dCY_lef/2

== system F16_dynamic_model_2019a/MODEL/Aerodynamic Forces and Moments on Body/Y-axis force coeff/dCY_da20 ==
  AoA : Inport
  beta : Inport  Port=2
  Add : Sum  Inputs=+-
  CY : Lookup_n-D  BreakpointsForDimension1=f16data.alpha1  BreakpointsForDimension2=f16data.beta  BreakpointsForDimension3=[5, 7]  Table=f16data.CY  ExtrapMethod=Clip  InternalRulePriority=Speed  RndMeth=Simplest
      settings: InputPortMap=u0,u1
  CY_da20 : Lookup_n-D  BreakpointsForDimension1=f16data.alpha1  BreakpointsForDimension2=f16data.beta  BreakpointsForDimension3=[5, 7]  Table=f16data.CY_da20  ExtrapMethod=Clip  InternalRulePriority=Speed  RndMeth=Simplest
      settings: InputPortMap=u0,u1
  CY_da20 - CY : Outport
  wires:
  AoA/1 -> CY/1, CY_da20/1
  beta/1 -> CY/2, CY_da20/2
  CY_da20/1 -> Add/1
  CY/1 -> Add/2
  Add/1 -> CY_da20 - CY/1

== system F16_dynamic_model_2019a/MODEL/Aerodynamic Forces and Moments on Body/Y-axis force coeff/dCY_da20_lef ==
  AoA : Inport
  "Sideslip " : Inport  Port=2
  dlef : Inport  Port=3
  Add : Sum  Inputs=+-
  CY : Lookup_n-D  BreakpointsForDimension1=f16data.alpha2  BreakpointsForDimension2=f16data.beta  BreakpointsForDimension3=[5, 7]  Table=f16data.CY_lef  ExtrapMethod=Clip  InternalRulePriority=Speed  RndMeth=Simplest
      settings: InputPortMap=u0,u1
  CY_da20 : Lookup_n-D  BreakpointsForDimension1=f16data.alpha1  BreakpointsForDimension2=f16data.beta  BreakpointsForDimension3=[5, 7]  Table=f16data.CY_da20  ExtrapMethod=Clip  InternalRulePriority=Speed  RndMeth=Simplest
      settings: InputPortMap=u0,u1
  CY_da20lef : Lookup_n-D  BreakpointsForDimension1=f16data.alpha2  BreakpointsForDimension2=f16data.beta  BreakpointsForDimension3=[5, 7]  Table=f16data.CY_da20lef  ExtrapMethod=Clip  InternalRulePriority=Speed  RndMeth=Simplest
      settings: InputPortMap=u0,u1
  Constant : Constant
  Multiply : Gain  Gain=1/(25)
  Product : Product
  Sum : Sum  Inputs=+-
  dCY_da20lef : Sum  Inputs=+--
  n-D Lookup Table : Lookup_n-D  BreakpointsForDimension1=f16data.alpha1  BreakpointsForDimension2=f16data.beta  BreakpointsForDimension3=[5, 7]  Table=f16data.CY  ExtrapMethod=Clip  InternalRulePriority=Speed  RndMeth=Simplest
      settings: InputPortMap=u0,u1
  dCY_da20lef * (1-dlef/25) : Outport
  wires:
  "Sideslip "/1 -> n-D Lookup Table/2, CY_da20/2, CY/2, CY_da20lef/2
  AoA/1 -> n-D Lookup Table/1, CY_da20/1, CY/1, CY_da20lef/1
  Constant/1 -> Sum/1
  CY/1 -> dCY_da20lef/2
  dlef/1 -> Multiply/1
  Multiply/1 -> Sum/2
  dCY_da20lef/1 -> Product/1
  Product/1 -> dCY_da20lef * (1-dlef/25)/1
  CY_da20lef/1 -> dCY_da20lef/1
  Sum/1 -> Product/2
  CY_da20/1 -> Add/1
  n-D Lookup Table/1 -> Add/2
  Add/1 -> dCY_da20lef/3

== system F16_dynamic_model_2019a/MODEL/Aerodynamic Forces and Moments on Body/Y-axis force coeff/dCY_dr30 ==
  AoA : Inport
  beta : Inport  Port=2
  Add : Sum  Inputs=+-
  CY : Lookup_n-D  BreakpointsForDimension1=f16data.alpha1  BreakpointsForDimension2=f16data.beta  BreakpointsForDimension3=[5, 7]  Table=f16data.CY  ExtrapMethod=Clip  InternalRulePriority=Speed  RndMeth=Simplest
      settings: InputPortMap=u0,u1
  CY_dr30 : Lookup_n-D  BreakpointsForDimension1=f16data.alpha1  BreakpointsForDimension2=f16data.beta  BreakpointsForDimension3=[5, 7]  Table=f16data.CY_dr30  ExtrapMethod=Clip  InternalRulePriority=Speed  RndMeth=Simplest
      settings: InputPortMap=u0,u1
  CY_dr30 - CY : Outport
  wires:
  CY_dr30/1 -> Add/1
  beta/1 -> CY/2, CY_dr30/2
  AoA/1 -> CY/1, CY_dr30/1
  CY/1 -> Add/2
  Add/1 -> CY_dr30 - CY/1

== system F16_dynamic_model_2019a/MODEL/Aerodynamic Forces and Moments on Body/Y-axis force coeff/dCYp_lef ==
  AoA : Inport
  dlef : Inport  Port=2
  Constant : Constant
  Multiply : Gain  Gain=1/(25)
  Product : Product
  Sum : Sum  Inputs=+-
  dCYp_lef : Lookup_n-D  NumberOfTableDimensions=1  BreakpointsForDimension1=f16data.alpha2  BreakpointsForDimension3=[5, 7]  Table=f16data.dCYp_lef  ExtrapMethod=Clip  InternalRulePriority=Speed  RndMeth=Simplest
  dCYp_lef * (1-dlef/25) : Outport
  wires:
  AoA/1 -> dCYp_lef/1
  Constant/1 -> Sum/1
  dlef/1 -> Multiply/1
  Multiply/1 -> Sum/2
  Product/1 -> dCYp_lef * (1-dlef/25)/1
  Sum/1 -> Product/2
  dCYp_lef/1 -> Product/1

== system F16_dynamic_model_2019a/MODEL/Aerodynamic Forces and Moments on Body/Y-axis force coeff/dCYr_lef ==
  AoA : Inport
  dlef : Inport  Port=2
  Constant : Constant
  Multiply : Gain  Gain=1/(25)
  Product : Product
  Sum : Sum  Inputs=+-
  dCYr_lef : Lookup_n-D  NumberOfTableDimensions=1  BreakpointsForDimension1=f16data.alpha2  BreakpointsForDimension3=[5, 7]  Table=f16data.dCYr_lef  ExtrapMethod=Clip  InternalRulePriority=Speed  RndMeth=Simplest
  dCYr_lef * (1-dlef/25) : Outport
  wires:
  AoA/1 -> dCYr_lef/1
  Constant/1 -> Sum/1
  dlef/1 -> Multiply/1
  Multiply/1 -> Sum/2
  Product/1 -> dCYr_lef * (1-dlef/25)/1
  Sum/1 -> Product/2
  dCYr_lef/1 -> Product/1

== system F16_dynamic_model_2019a/MODEL/Aerodynamic Forces and Moments on Body/Yawing-moment coeff/Cn ==
  AoA : Inport
  "beta " : Inport  Port=2
  dh : Inport  Port=3
  Cn table : Lookup_n-D  NumberOfTableDimensions=3  BreakpointsForDimension1=f16data.alpha1  BreakpointsForDimension2=f16data.beta  BreakpointsForDimension3=f16data.de2  Table=f16data.Cn  ExtrapMethod=Clip  InternalRulePriority=Speed  RndMeth=Simplest
      settings: InputPortMap=u0,u1,u2
  Cn : Outport
  wires:
  AoA/1 -> Cn table/1
  "beta "/1 -> Cn table/2
  dh/1 -> Cn table/3
  Cn table/1 -> Cn/1

== system F16_dynamic_model_2019a/MODEL/Aerodynamic Forces and Moments on Body/Yawing-moment coeff/Cnp ==
  AoA : Inport
  Cnp : Lookup_n-D  NumberOfTableDimensions=1  BreakpointsForDimension1=f16data.alpha1  BreakpointsForDimension3=[5, 7]  Table=f16data.Cnp  ExtrapMethod=Clip  InternalRulePriority=Speed  RndMeth=Simplest
  "Cnp " : Outport
  wires:
  AoA/1 -> Cnp/1
  Cnp/1 -> "Cnp "/1

== system F16_dynamic_model_2019a/MODEL/Aerodynamic Forces and Moments on Body/Yawing-moment coeff/Cnr ==
  AoA : Inport
  n-D Lookup Table : Lookup_n-D  NumberOfTableDimensions=1  BreakpointsForDimension1=f16data.alpha1  BreakpointsForDimension3=[5, 7]  Table=f16data.Cnr  ExtrapMethod=Clip  InternalRulePriority=Speed  RndMeth=Simplest
  Cnr : Outport
  wires:
  AoA/1 -> n-D Lookup Table/1
  n-D Lookup Table/1 -> Cnr/1

== system F16_dynamic_model_2019a/MODEL/Aerodynamic Forces and Moments on Body/Yawing-moment coeff/dCn_da20 ==
  AoA : Inport
  beta : Inport  Port=2
  dh : Inport  Port=3
  Add : Sum  Inputs=+-
  Cn : Lookup_n-D  NumberOfTableDimensions=3  BreakpointsForDimension1=f16data.alpha1  BreakpointsForDimension2=f16data.beta  BreakpointsForDimension3=f16data.de2  Table=f16data.Cn  ExtrapMethod=Clip  InternalRulePriority=Speed  RndMeth=Simplest
      settings: InputPortMap=u0,u1,u2
  Cn_da20 : Lookup_n-D  BreakpointsForDimension1=f16data.alpha1  BreakpointsForDimension2=f16data.beta  BreakpointsForDimension3=[5, 7]  Table=f16data.Cn_da20  ExtrapMethod=Clip  InternalRulePriority=Speed  RndMeth=Simplest
      settings: InputPortMap=u0,u1
  Multiply : Gain  Gain=0
  Cn_da20 - Cn : Outport
  wires:
  AoA/1 -> Cn/1, Cn_da20/1
  beta/1 -> Cn/2, Cn_da20/2
  Cn_da20/1 -> Add/1
  Cn/1 -> Add/2
  Add/1 -> Cn_da20 - Cn/1
  dh/1 -> Multiply/1
  Multiply/1 -> Cn/3

== system F16_dynamic_model_2019a/MODEL/Aerodynamic Forces and Moments on Body/Yawing-moment coeff/dCn_da20_lef ==
  AoA : Inport
  "Sideslip " : Inport  Port=2
  dlef : Inport  Port=3
  dh : Inport  Port=4
  Add : Sum  Inputs=+-
  Cn : Lookup_n-D  BreakpointsForDimension1=f16data.alpha2  BreakpointsForDimension2=f16data.beta  BreakpointsForDimension3=[5, 7]  Table=f16data.Cn_lef  ExtrapMethod=Clip  InternalRulePriority=Speed  RndMeth=Simplest
      settings: InputPortMap=u0,u1
  Cn table : Lookup_n-D  NumberOfTableDimensions=3  BreakpointsForDimension1=f16data.alpha1  BreakpointsForDimension2=f16data.beta  BreakpointsForDimension3=f16data.de2  Table=f16data.Cn  ExtrapMethod=Clip  InternalRulePriority=Speed  RndMeth=Simplest
      settings: InputPortMap=u0,u1,u2
  Cn_da20 : Lookup_n-D  BreakpointsForDimension1=f16data.alpha1  BreakpointsForDimension2=f16data.beta  BreakpointsForDimension3=[5, 7]  Table=f16data.Cn_da20  ExtrapMethod=Clip  InternalRulePriority=Speed  RndMeth=Simplest
      settings: InputPortMap=u0,u1
  Cn_da20lef : Lookup_n-D  BreakpointsForDimension1=f16data.alpha2  BreakpointsForDimension2=f16data.beta  BreakpointsForDimension3=[5, 7]  Table=f16data.Cn_da20lef  ExtrapMethod=Clip  InternalRulePriority=Speed  RndMeth=Simplest
      settings: InputPortMap=u0,u1
  Constant : Constant
  Multiply : Gain  Gain=1/(25)
  Multiply1 : Gain  Gain=0
  Product : Product
  Sum : Sum  Inputs=+-
  dCn_da20lef : Sum  Inputs=+--
  dCn_da20lef * (1-dlef/25) : Outport
  wires:
  "Sideslip "/1 -> Cn table/2, Cn_da20/2, Cn/2, Cn_da20lef/2
  AoA/1 -> Cn table/1, Cn_da20/1, Cn/1, Cn_da20lef/1
  Constant/1 -> Sum/1
  Cn/1 -> dCn_da20lef/2
  dlef/1 -> Multiply/1
  Multiply/1 -> Sum/2
  dCn_da20lef/1 -> Product/1
  Product/1 -> dCn_da20lef * (1-dlef/25)/1
  Cn_da20lef/1 -> dCn_da20lef/1
  Sum/1 -> Product/2
  Cn_da20/1 -> Add/1
  Cn table/1 -> Add/2
  Add/1 -> dCn_da20lef/3
  dh/1 -> Multiply1/1
  Multiply1/1 -> Cn table/3

== system F16_dynamic_model_2019a/MODEL/Aerodynamic Forces and Moments on Body/Yawing-moment coeff/dCn_dr30 ==
  AoA : Inport
  beta : Inport  Port=2
  dh : Inport  Port=3
  Add : Sum  Inputs=+-
  Cn_dr30 : Lookup_n-D  BreakpointsForDimension1=f16data.alpha1  BreakpointsForDimension2=f16data.beta  BreakpointsForDimension3=[5, 7]  Table=f16data.Cn_dr30  ExtrapMethod=Clip  InternalRulePriority=Speed  RndMeth=Simplest
      settings: InputPortMap=u0,u1
  Multiply : Gain  Gain=0
  n-D Lookup Table : Lookup_n-D  NumberOfTableDimensions=3  BreakpointsForDimension1=f16data.alpha1  BreakpointsForDimension2=f16data.beta  BreakpointsForDimension3=f16data.de2  Table=f16data.Cn  ExtrapMethod=Clip  InternalRulePriority=Speed  RndMeth=Simplest
      settings: InputPortMap=u0,u1,u2
  dCn_dr30 : Outport
  wires:
  Cn_dr30/1 -> Add/1
  dh/1 -> Multiply/1
  AoA/1 -> n-D Lookup Table/1, Cn_dr30/1
  Add/1 -> dCn_dr30/1
  n-D Lookup Table/1 -> Add/2
  beta/1 -> Cn_dr30/2, n-D Lookup Table/2
  Multiply/1 -> n-D Lookup Table/3

== system F16_dynamic_model_2019a/MODEL/Aerodynamic Forces and Moments on Body/Yawing-moment coeff/dCn_lef katsayılı terimi ==
  AoA : Inport
  beta : Inport  Port=2
  dh : Inport  Port=3
  dlef : Inport  Port=4
  Add : Sum  Inputs=+-
  Cn_lef : Lookup_n-D  BreakpointsForDimension1=f16data.alpha2  BreakpointsForDimension2=f16data.beta  BreakpointsForDimension3=[5, 7]  Table=f16data.Cn_lef  ExtrapMethod=Clip  InternalRulePriority=Speed  RndMeth=Simplest
      settings: InputPortMap=u0,u1
  Constant : Constant
  Multiply : Gain  Gain=0
  Multiply1 : Gain  Gain=1/(25)
  Product : Product
  Sum : Sum  Inputs=+-
  n-D Lookup Table : Lookup_n-D  NumberOfTableDimensions=3  BreakpointsForDimension1=f16data.alpha1  BreakpointsForDimension2=f16data.beta  BreakpointsForDimension3=f16data.de2  Table=f16data.Cn  ExtrapMethod=Clip  InternalRulePriority=Speed  RndMeth=Simplest
      settings: InputPortMap=u0,u1,u2
  dCn_lef * (1-dlef/25) : Outport
  wires:
  AoA/1 -> n-D Lookup Table/1, Cn_lef/1
  beta/1 -> Cn_lef/2, n-D Lookup Table/2
  dh/1 -> Multiply/1
  Multiply/1 -> n-D Lookup Table/3
  Cn_lef/1 -> Add/1
  n-D Lookup Table/1 -> Add/2
  Constant/1 -> Sum/1
  Multiply1/1 -> Sum/2
  Sum/1 -> Product/2
  dlef/1 -> Multiply1/1
  Add/1 -> Product/1
  Product/1 -> dCn_lef * (1-dlef/25)/1

== system F16_dynamic_model_2019a/MODEL/Aerodynamic Forces and Moments on Body/Yawing-moment coeff/dCnbeta ==
  AoA : Inport
  n-D Lookup Table : Lookup_n-D  NumberOfTableDimensions=1  BreakpointsForDimension1=f16data.alpha1  BreakpointsForDimension3=[5, 7]  Table=f16data.dCnbeta  ExtrapMethod=Clip  InternalRulePriority=Speed  RndMeth=Simplest
  "dCnbeta " : Outport
  wires:
  AoA/1 -> n-D Lookup Table/1
  n-D Lookup Table/1 -> "dCnbeta "/1

== system F16_dynamic_model_2019a/MODEL/Aerodynamic Forces and Moments on Body/Yawing-moment coeff/dCnp_lef ==
  AoA : Inport
  dlef : Inport  Port=2
  Constant : Constant
  Multiply : Gain  Gain=1/(25)
  Product : Product
  Sum : Sum  Inputs=+-
  dCnp_lef : Lookup_n-D  NumberOfTableDimensions=1  BreakpointsForDimension1=f16data.alpha2  BreakpointsForDimension3=[5, 7]  Table=f16data.dCnp_lef  ExtrapMethod=Clip  InternalRulePriority=Speed  RndMeth=Simplest
  dCnp_lef * (1-dlef/25) : Outport
  wires:
  AoA/1 -> dCnp_lef/1
  Constant/1 -> Sum/1
  dlef/1 -> Multiply/1
  Multiply/1 -> Sum/2
  Product/1 -> dCnp_lef * (1-dlef/25)/1
  Sum/1 -> Product/2
  dCnp_lef/1 -> Product/1

== system F16_dynamic_model_2019a/MODEL/Aerodynamic Forces and Moments on Body/Yawing-moment coeff/dCnr_lef ==
  AoA : Inport
  dlef : Inport  Port=2
  Constant : Constant
  Multiply : Gain  Gain=1/(25)
  Product : Product
  Sum : Sum  Inputs=+-
  dCnr_lef : Lookup_n-D  NumberOfTableDimensions=1  BreakpointsForDimension1=f16data.alpha2  BreakpointsForDimension3=[5, 7]  Table=f16data.dCnr_lef  ExtrapMethod=Clip  InternalRulePriority=Speed  RndMeth=Simplest
  dCnr_lef * (1-dlef/25) : Outport
  wires:
  AoA/1 -> dCnr_lef/1
  Constant/1 -> Sum/1
  dlef/1 -> Multiply/1
  Multiply/1 -> Sum/2
  Product/1 -> dCnr_lef * (1-dlef/25)/1
  Sum/1 -> Product/2
  dCnr_lef/1 -> Product/1

== system F16_dynamic_model_2019a/MODEL/Aerodynamic Forces and Moments on Body/Z-axis force coeff/CZ_q + dCZ_qlef ==
  AoA : Inport
  dlef : Inport  Port=2
  Add : Sum
  CZq : Lookup_n-D  NumberOfTableDimensions=1  BreakpointsForDimension1=f16data.alpha1  BreakpointsForDimension3=[5, 7]  Table=f16data.CZq  ExtrapMethod=Clip  InternalRulePriority=Speed  RndMeth=Simplest
  Constant : Constant
  Display : Display
  Display1 : Display
  Multiply : Gain  Gain=1/25
  Product : Product
  Sum : Sum  Inputs=+-
  dCZq_lef : Lookup_n-D  NumberOfTableDimensions=1  BreakpointsForDimension1=f16data.alpha2  BreakpointsForDimension3=[5, 7]  Table=f16data.dCZq_lef  ExtrapMethod=Clip  InternalRulePriority=Speed  RndMeth=Simplest
  Out1 : Outport
  wires:
  Add/1 -> Out1/1
  dCZq_lef/1 -> Display1/1, Product/1
  AoA/1 -> dCZq_lef/1, CZq/1
  Product/1 -> Add/2
  dlef/1 -> Multiply/1
  Sum/1 -> Product/2
  Constant/1 -> Sum/1
  Multiply/1 -> Sum/2
  CZq/1 -> Display/1, Add/1

== system F16_dynamic_model_2019a/MODEL/Aerodynamic Forces and Moments on Body/Z-axis force coeff/Subsystem ==
  AoA : Inport
  Sideslip : Inport  Port=2
  dh : Inport  Port=3
  CZ : Lookup_n-D  NumberOfTableDimensions=3  BreakpointsForDimension1=f16data.alpha1  BreakpointsForDimension2=f16data.beta  BreakpointsForDimension3=f16data.de1  Table=f16data.CZ  ExtrapMethod=Clip  InternalRulePriority=Speed  RndMeth=Simplest
      settings: InputPortMap=u0,u1,u2
  Cz : Outport
  wires:
  CZ/1 -> Cz/1
  AoA/1 -> CZ/1
  Sideslip/1 -> CZ/2
  dh/1 -> CZ/3

== system F16_dynamic_model_2019a/MODEL/Aerodynamic Forces and Moments on Body/Z-axis force coeff/dCZ, lef olan tüm terim ==
  AoA : Inport
  "Sideslip " : Inport  Port=2
  dh : Inport  Port=3
  dlef : Inport  Port=4
  CZ : Lookup_n-D  NumberOfTableDimensions=3  BreakpointsForDimension1=f16data.alpha1  BreakpointsForDimension2=f16data.beta  BreakpointsForDimension3=f16data.de1  Table=f16data.CZ  ExtrapMethod=Clip  InternalRulePriority=Speed  RndMeth=Simplest
      settings: InputPortMap=u0,u1,u2
  CZ_lef : Lookup_n-D  BreakpointsForDimension1=f16data.alpha2  BreakpointsForDimension2=f16data.beta  BreakpointsForDimension3=[5, 7]  Table=f16data.CZ_lef  ExtrapMethod=Clip  InternalRulePriority=Speed  RndMeth=Simplest
      settings: InputPortMap=u0,u1
  Constant : Constant
  Multiply : Gain  Gain=1/(25)
  Multiply1 : Gain  Gain=0
  Product : Product
  Sum : Sum  Inputs=+-
  dcz,lef : Sum  Inputs=+-
  dzx,lef * (1-dlef/25) : Outport
  wires:
  "Sideslip "/1 -> CZ/2, CZ_lef/2
  AoA/1 -> CZ/1, CZ_lef/1
  Product/1 -> dzx,lef * (1-dlef/25)/1
  dcz,lef/1 -> Product/1
  dh/1 -> Multiply1/1
  CZ_lef/1 -> dcz,lef/1
  CZ/1 -> dcz,lef/2
  Sum/1 -> Product/2
  Constant/1 -> Sum/1
  Multiply/1 -> Sum/2
  dlef/1 -> Multiply/1
  Multiply1/1 -> CZ/3

== system F16_dynamic_model_2019a/MODEL/Aerodynamic Forces and Moments on Body/Z-axis force coeff/dCZ_sb ==
  AoA : Inport
  dsb : Inport  Port=2
  Multiply : Gain  Gain=1/60
  Product : Product
  n-D Lookup Table : Lookup_n-D  NumberOfTableDimensions=1  BreakpointsForDimension1=f16data.alpha1  BreakpointsForDimension3=[5, 7]  Table=f16data.dCZ_sb  ExtrapMethod=Clip  InternalRulePriority=Speed  RndMeth=Simplest
  Out1 : Outport
  wires:
  dsb/1 -> Multiply/1
  AoA/1 -> n-D Lookup Table/1
  n-D Lookup Table/1 -> Product/1
  Multiply/1 -> Product/2
  Product/1 -> Out1/1

== system F16_dynamic_model_2019a/MODEL/Thrust on Body /Subsystem/Subsystem ==
  mil : Inport
  "max " : Inport  Port=2
  power : Inport  Port=3
  Add : Sum  Inputs=+-
  Add1 : Sum
  Add2 : Sum  Inputs=+-
  Constant : Constant  Value=50
  Constant1 : Constant  Value=50
  Product : Product
  Product1 : Product  Inputs=*/
  T : Outport
  wires:
  "max "/1 -> Add/1
  mil/1 -> Add1/1, Add/2
  Add1/1 -> T/1
  power/1 -> Add2/1
  Constant/1 -> Add2/2
  Add/1 -> Product/1
  Add2/1 -> Product/2
  Product/1 -> Product1/1
  Constant1/1 -> Product1/2
  Product1/1 -> Add1/2

== system F16_dynamic_model_2019a/MODEL/Thrust on Body /Subsystem/Subsystem1 ==
  "Mil " : Inport
  Idle : Inport  Port=2
  Power : Inport  Port=3
  Add : Sum  Inputs=+-
  Add1 : Sum
  Constant : Constant  Value=50
  Display : Display
  Product : Product  Inputs=*/
  Product1 : Product
  T : Outport
  wires:
  "Mil "/1 -> Add/1
  Idle/1 -> Add/2, Add1/1
  Power/1 -> Display/1, Product/1
  Constant/1 -> Product/2
  Add/1 -> Product1/1
  Product/1 -> Product1/2
  Product1/1 -> Add1/2
  Add1/1 -> T/1

== matlab function F16_dynamic_model_2019a/Altitude Hold/MATLAB Function ==
  settings: updateMethod=DISCRETE
  data: altitude_input input; altitude_output output; button_pressed input
function altitude_output  = store_and_return_altitude(altitude_input, button_pressed)
    % store_and_return_altitude - Tuşa basıldığında irtifa değerini kaydedip,
    % tekrar basana kadar o değeri çıktı olarak verir.

    % Global değişkeni tanımla (değeri kaydetmek için)
    persistent stored_altitude
    
    if isempty(stored_altitude)
        stored_altitude = NaN; % İlk başta saklanan değer yok
    end
    
    % Eğer tuşa basıldığında, irtifa kaydedecek
    if button_pressed
        stored_altitude = altitude_input;
    end
    
    % Kaydedilen irtifa değerini çıktı olarak ver
    altitude_output = stored_altitude;
end

== matlab function F16_dynamic_model_2019a/Altitude Hold/MATLAB Function2 ==
  data: button input; ahCheck output
function ahCheck = toggle(button)
% toggle: Butona basıldığında turn_check değerini 1 ve 0 arasında değiştirir.

persistent ah_check; % turn_check değişkenini kalıcı hale getirir
if isempty(ah_check)
    ah_check = 0; % Başlangıçta 0 olarak ayarla
end

if button == 1 % Buton basılıysa
    ah_check = 1 - ah_check; % turn_check değerini değiştir
end

ahCheck = ah_check; % Çıkış değerini ayarla
end

== matlab function F16_dynamic_model_2019a/Altitude Hold/MATLAB Function1 ==
  data: button input; turnCheck output
function turnCheck = toggle(button)
% toggle: Butona basıldığında turn_check değerini 1 ve 0 arasında değiştirir.

persistent turn_check; % turn_check değişkenini kalıcı hale getirir
if isempty(turn_check)
    turn_check = 0; % Başlangıçta 0 olarak ayarla
end

if button == 1 % Buton basılıysa
    turn_check = 1 - turn_check; % turn_check değerini değiştir
end

turnCheck = turn_check; % Çıkış değerini ayarla
end
